simulink model "Quad2D"  (R2017b)
settings: Solver=VariableStepAuto  StartTime=0.0  StopTime=t_end  FixedStep=0.00333  RelTol=1e-3
values from neighbouring files (symbols this model uses):
  GyroFreq = 1/80    (= 0.0125)    [zConstantGainLanding.m]    (also in zFPS.m; zHorizontal.m; zScaling.m; zTakeoff.m)
  noiseSeed = [23341,346834,734234,0,12]    [scaling.m]
  q0 = [1,3,degtorad(0),0,0,0]'    [zConstantGainLanding.m]    (also in zFPS.m = [1,1,degtorad(0),0,0,0]'; zHorizontal.m = [1,2,degtorad(0),0,0,0]'; zScaling.m = [1,1,degtorad(0),0,0,0]'; zTakeoff.m = [1,1,degtorad(0),0,0,0]')
  triggerStopX = 0    [zConstantGainLanding.m]    (also in zFPS.m; zHorizontal.m; zScaling.m; zTakeoff.m)
  triggerStopZ = 0    [zConstantGainLanding.m]    (also in zFPS.m; zHorizontal.m; zScaling.m; zTakeoff.m)
undefined symbols (not defined in the file or in its folder): fps, Quad2D_control, Quad2D_eom
libraries: simulink x8
settings Model: Creator=titus  LastModifiedBy=titus
settings DataIOCC: SaveFormat=Array
settings DebuggingCC: AlgebraicLoopMsg=none
settings CodeAppCC: StateflowObjectComments=on

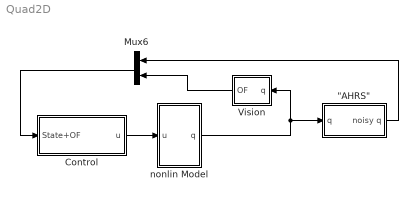
== system Quad2D ==
  "\"AHRS\"" : Subsystem
  Control : Subsystem
  Mux6 : Mux  Inputs=2
  Vision : Subsystem
  nonlin Model : Subsystem
  wires:
  Mux6/1 -> Control/1(State+OF)
  Control/1(u) -> nonlin Model/1(u)
  nonlin Model/1(q) -> Vision/1(q), "\"AHRS\""/1(q)
  "\"AHRS\""/1(noisy q) -> Mux6/1
  Vision/1(OF) -> Mux6/2

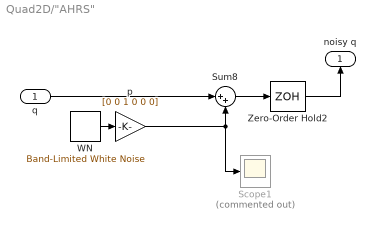
== system Quad2D/"AHRS" ==
  q : Inport
  Scope1 : Scope  Commented=on
  Sum8 : Sum  Inputs=|++
  WN : simulink/Sources/Band-Limited White Noise  Cov=GyroNoise  Ts=GyroFreq  seed=noiseSeed(3)
  Zero-Order Hold2 : ZeroOrderHold  SampleTime=1/512
  p : Gain  Gain=[0 0 1 0 0 0]
  noisy q : Outport
  wires:
  q/1 -> Sum8/1
  Sum8/1 -> Zero-Order Hold2/1
  WN/1 -> p/1
  p/1 -> Scope1/1, Sum8/2
  Zero-Order Hold2/1 -> noisy q/1

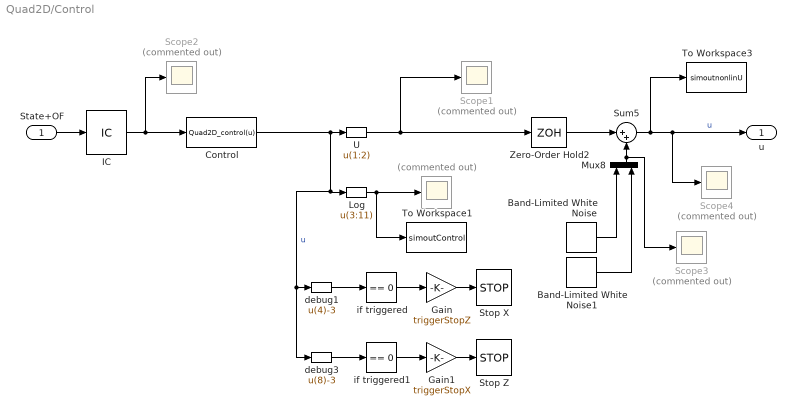
== system Quad2D/Control ==
  State+OF : Inport
  " " : Scope  Commented=on
  Band-Limited White Noise : simulink/Sources/Band-Limited White Noise  Cov=ActuatorNoise  Ts=0.2  seed=noiseSeed(1)
  Band-Limited White Noise1 : simulink/Sources/Band-Limited White Noise  Cov=ActuatorNoise  Ts=0.2  seed=noiseSeed(2)
  Control : MATLABFcn  InitFcn=clear Quad2D_control;  MATLABFcn=Quad2D_control(u)
  Gain : Gain  Gain=triggerStopZ  OutDataTypeStr=Inherit: Same as input
  Gain1 : Gain  Gain=triggerStopX  OutDataTypeStr=Inherit: Same as input
  IC : InitialCondition  Value=[q0;q0(4)/q0(2);q0(5)/q0(2)]
  Log : MATLABFcn  MATLABFcn=u(3:11)
  Mux8 : Mux  Inputs=2
  Scope{1..4} (4 alike) : Scope  Commented=on
  Stop X : Stop
  Stop Z : Stop
  Sum5 : Sum  Inputs=|++
  To Workspace1 : ToWorkspace  VariableName=simoutControl  SaveFormat=Timeseries  SampleTime=-1
  To Workspace3 : ToWorkspace  VariableName=simoutnonlinU  SaveFormat=Timeseries  SampleTime=-1
  U : MATLABFcn  MATLABFcn=u(1:2)
  Zero-Order Hold2 : ZeroOrderHold  SampleTime=1/512
  debug1 : MATLABFcn  MATLABFcn=u(4)-3
  debug3 : MATLABFcn  MATLABFcn=u(8)-3
  if triggered : simulink/Logic and Bit Operations/Compare To Zero  relop===  OutDataTypeStr=boolean
  if triggered1 : simulink/Logic and Bit Operations/Compare To Zero  relop===  OutDataTypeStr=boolean
  u : Outport
  wires:
  Sum5/1 -> To Workspace3/1, u/1, Scope4/1  "u"
  State+OF/1 -> IC/1
  Control/1 -> debug3/1, debug1/1, Log/1, U/1  "u"
  Mux8/1 -> Scope3/1, Sum5/2
  U/1 -> Zero-Order Hold2/1, Scope1/1
  Log/1 -> To Workspace1/1, " "/1
  debug1/1 -> if triggered/1
  if triggered/1 -> Gain/1
  Gain/1 -> Stop X/1
  debug3/1 -> if triggered1/1
  if triggered1/1 -> Gain1/1
  Gain1/1 -> Stop Z/1
  IC/1 -> Scope2/1, Control/1
  Zero-Order Hold2/1 -> Sum5/1
  Band-Limited White Noise/1 -> Mux8/1
  Band-Limited White Noise1/1 -> Mux8/2

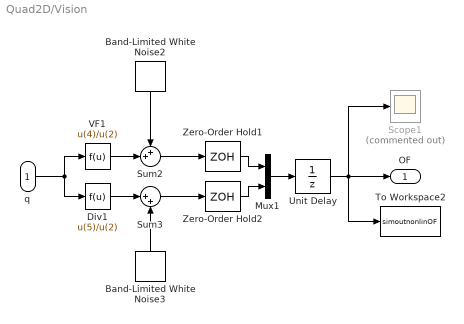
== system Quad2D/Vision ==
  q : Inport
  Band-Limited White Noise2 : simulink/Sources/Band-Limited White Noise  Cov=visionNoise  Ts=1/fps  seed=noiseSeed(4)
  Band-Limited White Noise3 : simulink/Sources/Band-Limited White Noise  Cov=visionNoise  Ts=1/fps  seed=noiseSeed(5)
  Div1 : Fcn  Expr=u(5)/u(2)
  Mux1 : Mux  Inputs=2
  Scope1 : Scope  Commented=on
  Sum2 : Sum  Inputs=++|
  Sum3 : Sum  Inputs=|++
  To Workspace2 : ToWorkspace  VariableName=simoutnonlinOF  SaveFormat=Timeseries  SampleTime=-1
  Unit Delay : UnitDelay  SampleTime=-1
  VF1 : Fcn  Expr=u(4)/u(2)
  Zero-Order Hold1 : ZeroOrderHold  SampleTime=1/fps
  Zero-Order Hold2 : ZeroOrderHold  SampleTime=1/fps
  OF : Outport
  wires:
  Sum3/1 -> Zero-Order Hold2/1
  Div1/1 -> Sum3/1
  Band-Limited White Noise3/1 -> Sum3/2
  q/1 -> VF1/1, Div1/1
  Unit Delay/1 -> Scope1/1, OF/1, To Workspace2/1
  Sum2/1 -> Zero-Order Hold1/1
  VF1/1 -> Sum2/2
  Band-Limited White Noise2/1 -> Sum2/1
  Zero-Order Hold1/1 -> Mux1/1
  Mux1/1 -> Unit Delay/1
  Zero-Order Hold2/1 -> Mux1/2

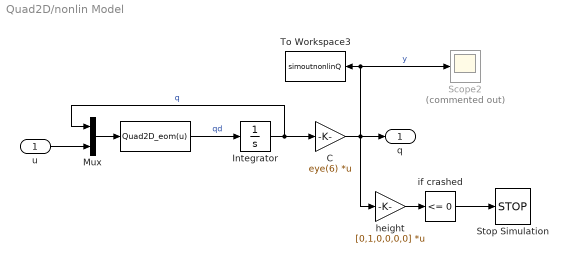
== system Quad2D/nonlin Model ==
  u : Inport
  " " : MATLABFcn  MATLABFcn=Quad2D_eom(u)
  C : Gain  Gain=eye(6)  Multiplication=Matrix(K*u)
  Integrator : Integrator  InitialCondition=q0
  Mux : Mux  Inputs=2
  Scope2 : Scope  Commented=on
  Stop Simulation : Stop
  To Workspace3 : ToWorkspace  VariableName=simoutnonlinQ  SaveFormat=Timeseries  SampleTime=-1
  height : Gain  Gain=[0,1,0,0,0,0]  Multiplication=Matrix(K*u)
  if crashed : simulink/Logic and Bit Operations/Compare To Zero  relop=<=  OutDataTypeStr=boolean
  q : Outport
  wires:
  Integrator/1 -> C/1, Mux/1  "q"
  Mux/1 -> " "/1
  C/1 -> height/1, q/1, Scope2/1, To Workspace3/1  "y"
  " "/1 -> Integrator/1  "qd"
  u/1 -> Mux/2
  height/1 -> if crashed/1
  if crashed/1 -> Stop Simulation/1
